simulink model "STEVE_Simulation"  (R2025b)
settings: Solver=ode8  StartTime=0  StopTime=300  FixedStep=0.0001  MaxStep=0.0001  RelTol=1e-3
model workspace (MAT data in the model file):
  op_trim1 = opcond.OperatingReport
  op_trim1.TerminationString_ = 'Operating point specifications were successfully met.'
  op_trim1.OptimizationOutput_.iterations = 3
  op_trim1.OptimizationOutput_.funcCount = 171
  op_trim1.OptimizationOutput_.lssteplength = 1
  op_trim1.OptimizationOutput_.stepsize = 4.63262973918e-09
  op_trim1.OptimizationOutput_.algorithm = 'active-set'
  op_trim1.OptimizationOutput_.firstorderopt = 2.40097601741e-08
  op_trim1.OptimizationOutput_.constrviolation = 8.47716769092e-07
  op_trim1.OptimizationOutput_.message = 'Local minimum found that satisfies the constraints.
    | 
    | Optimization completed because the objective function is non-decreasing in 
    | feasible directions, to within the value of the optimality tolerance,
    | and constraints are satisfied to within the  value of the constraint tolerance.
    | 
    | <stopping criteria details>
    | 
    | Optimization completed: The first-order optimality measure, 2.400976e-08, is less
    | than options.OptimalityTolerance = 1.000000e-06, and the maximum constraint violation,
    | 8.477168e-07,is less than options.ConstraintTolerance = 1.000000e-06.'
  op_trim1.OptimizationOutput_.bestfeasible.x = [4290.04874097; 10725.1258376; 15852.6764872; 0.313155746169; -0.0981866680343; -0.0652604980678; 0.0059055243257; -0.636615168463; 8.14642489212e-06; -0.0176940249338; -0.00155509692213; -9.31199930506e-05; -0.000181100785288; 15.418172162; 0.559389025394; 3.31048087203; -37.2767340788; 1.38336022573; 8.21403291962e-06; 8.22046546553e-06; 8.22180678664e-06; 8.18637735168e-06; 8.165374813e-06; 8.15659926853e-06; 8.21875394544e-06; 8.19540646323e-06; 8.20244331077e-06; 8.1953609355e-06; 8.1983838895e-06; 8.22592390188e-06; 8.20694393928e-06; 8.20085018843e-06; 8.25311843786e-06; 8.2421945992e-06; 4.99999832196; 1.99999584909; 1.99999585143; 4.99999832977; 1.99999587773; 1.999995897; -0.000340053296214]
  op_trim1.OptimizationOutput_.bestfeasible.fval = 0
  op_trim1.OptimizationOutput_.bestfeasible.constrviolation = 8.47716769092e-07
  op_trim1.OptimizationOutput_.bestfeasible.firstorderopt = 2.40097601741e-08
  op_trim1.OptimizationOutput_.progress = {'<font face="monospaced"; size=3><BR>', 'Optimizing to solve for all desired dx/dt=0, x(k+1)-x(k)=0, and y=ydes.<BR>', ' <BR>', '(Maximum Error)  Block<BR>', ' ---------------------------------------------------------<BR>', '(3.86548e-01) STEVE_Simulation/STeVe System Model/Vehicle Dynamics/3DOF to 6DOF/Custom Variable Mass 3dof (Body Axes)<BR>', '(3.86551e-01) STEVE_Simulation/STeVe System Model/Vehicle Dynamics/3DOF to 6DOF/Custom Variable Mass 3dof (Body Axes)<BR>', '(8.47360e-07) STEVE_Simulation/STeVe System Model/Vehicle Dynamics/3DOF to 6DOF/Custom Variable Mass 3dof (Body Axes)<BR>', '(8.47764e-07) STEVE_Simulation/STeVe System Model/Vehicle Dynamics/3DOF to 6DOF/Custom Variable Mass 3dof (Body Axes)<BR>', '(8.47764e-07) STEVE_Simulation/STeVe System Model/Vehicle Dynamics/3DOF to 6DOF/Custom Variable Mass 3dof (Body Axes)<BR>', ' <BR>', 'Operating point specifications were successfully met.<BR>'}
  op_trim1.Model_ = 'STEVE_Simulation'
  op_trim1.States_(1) = opcond.StateReport
  op_trim1.States_(1).Nx_ = 1
  op_trim1.States_(1).Block_ = 'STEVE_Simulation/Environment/Wind/Discrete Wind Gust Model/Distance into
    | gust (x)/Distance into
    | Gust (x)
    | (Limited to gust length d)'
  op_trim1.States_(1).x_ = 1.999995897
  op_trim1.States_(1).SteadyState_ = 0
  op_trim1.States_(1).dxMin_ = -Inf
  op_trim1.States_(1).dxMax_ = Inf
  op_trim1.States_(1).Known_ = 0
  op_trim1.States_(1).Min_ = 0
  op_trim1.States_(1).Max_ = 2
  op_trim1.States_(2) = opcond.StateReport
  op_trim1.States_(2).Nx_ = 1
  op_trim1.States_(2).Block_ = 'STEVE_Simulation/Environment/Wind/Discrete Wind Gust Model/Distance into
    | gust (y)/Distance into
    | Gust (x)
    | (Limited to gust length d)
    | '
  op_trim1.States_(2).x_ = 1.99999587773
  op_trim1.States_(2).SteadyState_ = 0
  op_trim1.States_(2).dxMin_ = -Inf
  op_trim1.States_(2).dxMax_ = Inf
  op_trim1.States_(2).Known_ = 0
  op_trim1.States_(2).Min_ = 0
  op_trim1.States_(2).Max_ = 2
  op_trim1.States_(3) = opcond.StateReport
  op_trim1.States_(3).Nx_ = 1
  op_trim1.States_(3).Block_ = 'STEVE_Simulation/Environment/Wind/Discrete Wind Gust Model/Distance into
    | gust (z)/Distance into
    | Gust (x)
    | (Limited to gust length d)
    | '
  op_trim1.States_(3).x_ = 4.99999832977
  op_trim1.States_(3).SteadyState_ = 0
  op_trim1.States_(3).dxMin_ = -Inf
  op_trim1.States_(3).dxMax_ = Inf
  op_trim1.States_(3).Known_ = 0
  op_trim1.States_(3).Min_ = 0
  op_trim1.States_(3).Max_ = 5
  op_trim1.States_(4) = opcond.StateReport
  op_trim1.States_(4).Nx_ = 1
  op_trim1.States_(4).Block_ = 'STEVE_Simulation/Environment/Wind/Discrete Wind Gust Model1/Distance into
    | gust (x)/Distance into
    | Gust (x)
    | (Limited to gust length d)'
  op_trim1.States_(4).x_ = 1.99999585143
  op_trim1.States_(4).SteadyState_ = 0
  op_trim1.States_(4).dxMin_ = -Inf
  op_trim1.States_(4).dxMax_ = Inf
  op_trim1.States_(4).Known_ = 0
  op_trim1.States_(4).Min_ = 0
  op_trim1.States_(4).Max_ = 2
  op_trim1.States_(5) = opcond.StateReport
  op_trim1.States_(5).Nx_ = 1
  op_trim1.States_(5).Block_ = 'STEVE_Simulation/Environment/Wind/Discrete Wind Gust Model1/Distance into
    | gust (y)/Distance into
    | Gust (x)
    | (Limited to gust length d)
    | '
  op_trim1.States_(5).x_ = 1.99999584909
  op_trim1.States_(5).SteadyState_ = 0
  op_trim1.States_(5).dxMin_ = -Inf
  op_trim1.States_(5).dxMax_ = Inf
  op_trim1.States_(5).Known_ = 0
  op_trim1.States_(5).Min_ = 0
  op_trim1.States_(5).Max_ = 2
  op_trim1.States_(6) = opcond.StateReport
  op_trim1.States_(6).Nx_ = 1
  op_trim1.States_(6).Block_ = 'STEVE_Simulation/Environment/Wind/Discrete Wind Gust Model1/Distance into
    | gust (z)/Distance into
    | Gust (x)
    | (Limited to gust length d)
    | '
  op_trim1.States_(6).x_ = 4.99999832196
  op_trim1.States_(6).SteadyState_ = 0
  op_trim1.States_(6).dxMin_ = -Inf
  op_trim1.States_(6).dxMax_ = Inf
  op_trim1.States_(6).Known_ = 0
  op_trim1.States_(6).Min_ = 0
  op_trim1.States_(6).Max_ = 5
  op_trim1.States_(7) = opcond.StateReport
  op_trim1.States_(7).dx_ = [0; 0]
  op_trim1.States_(7).Nx_ = 2
  op_trim1.States_(7).Block_ = 'STEVE_Simulation/Environment/Wind/Dryden Wind Turbulence Model 
    | (Continuous (+q +r))/Filters on angular rates/Hpgw/pgw_p'
  op_trim1.States_(7).x_ = [8.25311843786e-06; 8.2421945992e-06]
  op_trim1.States_(7).SteadyState_ = [0; 0]
  op_trim1.States_(7).dxMin_ = [-Inf; -Inf]
  op_trim1.States_(7).dxMax_ = [Inf; Inf]
  op_trim1.States_(7).Known_ = [0; 0]
  op_trim1.States_(7).Min_ = [-Inf; -Inf]
  op_trim1.States_(7).Max_ = [Inf; Inf]
  op_trim1.States_(8) = opcond.StateReport
  op_trim1.States_(8).dx_ = [0; 0]
  op_trim1.States_(8).Nx_ = 2
  op_trim1.States_(8).Block_ = 'STEVE_Simulation/Environment/Wind/Dryden Wind Turbulence Model 
    | (Continuous (+q +r))/Filters on angular rates/Hqgw/qgw_p'
  op_trim1.States_(8).x_ = [8.20694393928e-06; 8.20085018843e-06]
  op_trim1.States_(8).SteadyState_ = [0; 0]
  op_trim1.States_(8).dxMin_ = [-Inf; -Inf]
  op_trim1.States_(8).dxMax_ = [Inf; Inf]
  op_trim1.States_(8).Known_ = [0; 0]
  op_trim1.States_(8).Min_ = [-Inf; -Inf]
  op_trim1.States_(8).Max_ = [Inf; Inf]
  op_trim1.States_(9) = opcond.StateReport
  op_trim1.States_(9).dx_ = [0; 0]
  op_trim1.States_(9).Nx_ = 2
  op_trim1.States_(9).Block_ = 'STEVE_Simulation/Environment/Wind/Dryden Wind Turbulence Model 
    | (Continuous (+q +r))/Filters on angular rates/Hrgw/rgw_p'
  op_trim1.States_(9).x_ = [8.1983838895e-06; 8.22592390188e-06]
  op_trim1.States_(9).SteadyState_ = [0; 0]
  op_trim1.States_(9).dxMin_ = [-Inf; -Inf]
  op_trim1.States_(9).dxMax_ = [Inf; Inf]
  op_trim1.States_(9).Known_ = [0; 0]
  op_trim1.States_(9).Min_ = [-Inf; -Inf]
  op_trim1.States_(9).Max_ = [Inf; Inf]
  op_trim1.States_(10) = opcond.StateReport
  op_trim1.States_(10).dx_ = [0; 0]
  op_trim1.States_(10).Nx_ = 2
  op_trim1.States_(10).Block_ = 'STEVE_Simulation/Environment/Wind/Dryden Wind Turbulence Model 
    | (Continuous (+q +r))/Filters on velocities/Hugw(s)/ug_p'
  op_trim1.States_(10).x_ = [8.20244331077e-06; 8.1953609355e-06]
  op_trim1.States_(10).SteadyState_ = [0; 0]
  op_trim1.States_(10).dxMin_ = [-Inf; -Inf]
  op_trim1.States_(10).dxMax_ = [Inf; Inf]
  op_trim1.States_(10).Known_ = [0; 0]
  op_trim1.States_(10).Min_ = [-Inf; -Inf]
  op_trim1.States_(10).Max_ = [Inf; Inf]
  op_trim1.States_(11) = opcond.StateReport
  op_trim1.States_(11).dx_ = [0; 0]
  op_trim1.States_(11).Nx_ = 2
  op_trim1.States_(11).Block_ = 'STEVE_Simulation/Environment/Wind/Dryden Wind Turbulence Model 
    | (Continuous (+q +r))/Filters on velocities/Hvgw(s)/vg_p1'
  op_trim1.States_(11).x_ = [8.165374813e-06; 8.15659926853e-06]
  op_trim1.States_(11).SteadyState_ = [0; 0]
  op_trim1.States_(11).dxMin_ = [-Inf; -Inf]
  op_trim1.States_(11).dxMax_ = [Inf; Inf]
  op_trim1.States_(11).Known_ = [0; 0]
  op_trim1.States_(11).Min_ = [-Inf; -Inf]
  op_trim1.States_(11).Max_ = [Inf; Inf]
  op_trim1.States_(12) = opcond.StateReport
  op_trim1.States_(12).dx_ = [0; 0]
  op_trim1.States_(12).Nx_ = 2
  op_trim1.States_(12).Block_ = 'STEVE_Simulation/Environment/Wind/Dryden Wind Turbulence Model 
    | (Continuous (+q +r))/Filters on velocities/Hvgw(s)/vgw_p2'
  op_trim1.States_(12).x_ = [8.21875394544e-06; 8.19540646323e-06]
  op_trim1.States_(12).SteadyState_ = [0; 0]
  op_trim1.States_(12).dxMin_ = [-Inf; -Inf]
  op_trim1.States_(12).dxMax_ = [Inf; Inf]
  op_trim1.States_(12).Known_ = [0; 0]
  op_trim1.States_(12).Min_ = [-Inf; -Inf]
  op_trim1.States_(12).Max_ = [Inf; Inf]
  op_trim1.States_(13) = opcond.StateReport
  op_trim1.States_(13).dx_ = [0; 0]
  op_trim1.States_(13).Nx_ = 2
  op_trim1.States_(13).Block_ = 'STEVE_Simulation/Environment/Wind/Dryden Wind Turbulence Model 
    | (Continuous (+q +r))/Filters on velocities/Hwgw(s)/wg_p1'
  op_trim1.States_(13).x_ = [8.21403291962e-06; 8.22046546553e-06]
  op_trim1.States_(13).SteadyState_ = [0; 0]
  op_trim1.States_(13).dxMin_ = [-Inf; -Inf]
  op_trim1.States_(13).dxMax_ = [Inf; Inf]
  op_trim1.States_(13).Known_ = [0; 0]
  op_trim1.States_(13).Min_ = [-Inf; -Inf]
  op_trim1.States_(13).Max_ = [Inf; Inf]
  op_trim1.States_(14) = opcond.StateReport
  op_trim1.States_(14).dx_ = [0; 0]
  op_trim1.States_(14).Nx_ = 2
  op_trim1.States_(14).Block_ = 'STEVE_Simulation/Environment/Wind/Dryden Wind Turbulence Model 
    | (Continuous (+q +r))/Filters on velocities/Hwgw(s)/wg_p2'
  op_trim1.States_(14).x_ = [8.22180678664e-06; 8.18637735168e-06]
  op_trim1.States_(14).SteadyState_ = [0; 0]
  op_trim1.States_(14).dxMin_ = [-Inf; -Inf]
  op_trim1.States_(14).dxMax_ = [Inf; Inf]
  op_trim1.States_(14).Known_ = [0; 0]
  op_trim1.States_(14).Min_ = [-Inf; -Inf]
  op_trim1.States_(14).Max_ = [Inf; Inf]
  op_trim1.States_(15) = opcond.StateReport
  op_trim1.States_(15).dx_ = [-1624.62107391; 4290.04874097; 10725.1258376]
  op_trim1.States_(15).Nx_ = 3
  op_trim1.States_(15).Block_ = 'STEVE_Simulation/GuidanceCommands/Transfer Fcn'
  op_trim1.States_(15).x_ = [4290.04874097; 10725.1258376; 15852.6764872]
  op_trim1.States_(15).SteadyState_ = [0; 0; 0]
  op_trim1.States_(15).dxMin_ = [-Inf; -Inf; -Inf]
  op_trim1.States_(15).dxMax_ = [Inf; Inf; Inf]
  op_trim1.States_(15).Known_ = [0; 0; 0]
  op_trim1.States_(15).Min_ = [-Inf; -Inf; -Inf]
  op_trim1.States_(15).Max_ = [Inf; Inf; Inf]
  op_trim1.States_(16) = opcond.StateReport
  op_trim1.States_(16).dx_ = -3.37116243602
  op_trim1.States_(16).Nx_ = 1
  op_trim1.States_(16).Block_ = 'STEVE_Simulation/STeVe System Model/Control System/Classical Upgraded/PID Controller1/Filter/Cont. Filter/Filter'
  op_trim1.States_(16).x_ = -0.00155509692213
  op_trim1.States_(16).SteadyState_ = 0
  op_trim1.States_(16).dxMin_ = -Inf
  op_trim1.States_(16).dxMax_ = Inf
  op_trim1.States_(16).Known_ = 0
  op_trim1.States_(16).Min_ = -Inf
  op_trim1.States_(16).Max_ = Inf
  op_trim1.States_(17) = opcond.StateReport
  op_trim1.States_(17).dx_ = -0.00991390700733
  op_trim1.States_(17).Nx_ = 1
  op_trim1.States_(17).Block_ = 'STEVE_Simulation/STeVe System Model/Control System/Classical Upgraded/PID Controller1/Integrator/Continuous/Integrator'
  op_trim1.States_(17).x_ = -0.0176940249338
  op_trim1.States_(17).SteadyState_ = 0
  op_trim1.States_(17).dxMin_ = -Inf
  op_trim1.States_(17).dxMax_ = Inf
  op_trim1.States_(17).Known_ = 0
  op_trim1.States_(17).Min_ = -Inf
  op_trim1.States_(17).Max_ = Inf
  op_trim1.States_(18) = opcond.StateReport
  op_trim1.States_(18).dx_ = 0.00151513100245
  op_trim1.States_(18).Nx_ = 1
  op_trim1.States_(18).Block_ = 'STEVE_Simulation/STeVe System Model/Control System/Classical Upgraded/PID Controller2/Filter/Cont. Filter/Filter'
  op_trim1.States_(18).x_ = 0.0059055243257
  op_trim1.States_(18).SteadyState_ = 0
  op_trim1.States_(18).dxMin_ = -Inf
  op_trim1.States_(18).dxMax_ = Inf
  op_trim1.States_(18).Known_ = 0
  op_trim1.States_(18).Min_ = -Inf
  op_trim1.States_(18).Max_ = Inf
  op_trim1.States_(19) = opcond.StateReport
  op_trim1.States_(19).dx_ = -0.037481221471
  op_trim1.States_(19).Nx_ = 1
  op_trim1.States_(19).Block_ = 'STEVE_Simulation/STeVe System Model/Control System/Classical Upgraded/PID Controller2/Integrator/Continuous/Integrator'
  op_trim1.States_(19).x_ = -0.0652604980678
  op_trim1.States_(19).SteadyState_ = 0
  op_trim1.States_(19).dxMin_ = -Inf
  op_trim1.States_(19).dxMax_ = Inf
  op_trim1.States_(19).Known_ = 0
  op_trim1.States_(19).Min_ = -Inf
  op_trim1.States_(19).Max_ = Inf
  op_trim1.States_(20) = opcond.StateReport
  op_trim1.States_(20).dx_ = -0.0747869203805
  op_trim1.States_(20).Nx_ = 1
  op_trim1.States_(20).Block_ = 'STEVE_Simulation/STeVe System Model/Control System/Classical Upgraded/PID Controller3/Filter/Cont. Filter/Filter'
  op_trim1.States_(20).x_ = -0.0981866680343
  op_trim1.States_(20).SteadyState_ = 0
  op_trim1.States_(20).dxMin_ = -Inf
  op_trim1.States_(20).dxMax_ = Inf
  op_trim1.States_(20).Known_ = 0
  op_trim1.States_(20).Min_ = -Inf
  op_trim1.States_(20).Max_ = Inf
  op_trim1.States_(21) = opcond.StateReport
  op_trim1.States_(21).dx_ = 0.273198142244
  op_trim1.States_(21).Nx_ = 1
  op_trim1.States_(21).Block_ = 'STEVE_Simulation/STeVe System Model/Control System/Classical Upgraded/PID Controller3/Integrator/Continuous/Integrator'
  op_trim1.States_(21).x_ = 0.313155746169
  op_trim1.States_(21).SteadyState_ = 0
  op_trim1.States_(21).dxMin_ = -Inf
  op_trim1.States_(21).dxMax_ = Inf
  op_trim1.States_(21).Known_ = 0
  op_trim1.States_(21).Min_ = -Inf
  op_trim1.States_(21).Max_ = Inf
  op_trim1.States_(22) = opcond.StateReport
  op_trim1.States_(22).dx_ = -0.000814642489212
  op_trim1.States_(22).Nx_ = 1
  op_trim1.States_(22).Block_ = 'STEVE_Simulation/STeVe System Model/Control System/Classical Upgraded/PID Controller6/Filter/Cont. Filter/Filter'
  op_trim1.States_(22).x_ = 8.14642489212e-06
  op_trim1.States_(22).SteadyState_ = 0
  op_trim1.States_(22).dxMin_ = -Inf
  op_trim1.States_(22).dxMax_ = Inf
  op_trim1.States_(22).Known_ = 0
  op_trim1.States_(22).Min_ = -Inf
  op_trim1.States_(22).Max_ = Inf
  op_trim1.States_(23) = opcond.StateReport
  op_trim1.States_(23).dx_ = -0.133481022202
  op_trim1.States_(23).Nx_ = 1
  op_trim1.States_(23).Block_ = 'STEVE_Simulation/STeVe System Model/Control System/Classical Upgraded/PID Controller6/Integrator/Continuous/Integrator'
  op_trim1.States_(23).x_ = -0.636615168463
  op_trim1.States_(23).SteadyState_ = 0
  op_trim1.States_(23).dxMin_ = -Inf
  op_trim1.States_(23).dxMax_ = Inf
  op_trim1.States_(23).Known_ = 0
  op_trim1.States_(23).Min_ = -Inf
  op_trim1.States_(23).Max_ = Inf
  op_trim1.States_(24) = opcond.StateReport
  op_trim1.States_(24).dx_ = 3.05199662227
  op_trim1.States_(24).Nx_ = 1
  op_trim1.States_(24).Block_ = 'STEVE_Simulation/STeVe System Model/Vehicle Dynamics/3DOF to 6DOF/Custom Variable Mass 3dof
    | (Body Axes)'
  op_trim1.States_(24).StateName_ = 'u'
  op_trim1.States_(24).x_ = 15.418172162
  op_trim1.States_(24).SteadyState_ = 0
  op_trim1.States_(24).dxMin_ = -Inf
  op_trim1.States_(24).dxMax_ = Inf
  op_trim1.States_(24).Known_ = 0
  op_trim1.States_(24).Min_ = -Inf
  op_trim1.States_(24).Max_ = Inf
  op_trim1.States_(25) = opcond.StateReport
  op_trim1.States_(25).dx_ = 1.82984252685
  op_trim1.States_(25).Nx_ = 1
  op_trim1.States_(25).Block_ = 'STEVE_Simulation/STeVe System Model/Vehicle Dynamics/3DOF to 6DOF/Custom Variable Mass 3dof
    | (Body Axes)'
  op_trim1.States_(25).StateName_ = 'w'
  op_trim1.States_(25).x_ = 0.559389025394
  op_trim1.States_(25).SteadyState_ = 0
  op_trim1.States_(25).dxMin_ = -Inf
  op_trim1.States_(25).dxMax_ = Inf
  op_trim1.States_(25).Known_ = 0
  op_trim1.States_(25).Min_ = -Inf
  op_trim1.States_(25).Max_ = Inf
  op_trim1.States_(26) = opcond.StateReport
  op_trim1.States_(26).dx_ = 3.42262162857
  op_trim1.States_(26).Nx_ = 1
  op_trim1.States_(26).Block_ = 'STEVE_Simulation/STeVe System Model/Vehicle Dynamics/3DOF to 6DOF/Custom Variable Mass 3dof
    | (Body Axes)'
  op_trim1.States_(26).StateName_ = 'Xe'
  op_trim1.States_(26).x_ = 3.31048087203
  op_trim1.States_(26).SteadyState_ = 0
  op_trim1.States_(26).dxMin_ = -Inf
  op_trim1.States_(26).dxMax_ = Inf
  op_trim1.States_(26).Known_ = 0
  op_trim1.States_(26).Min_ = -Inf
  op_trim1.States_(26).Max_ = Inf
  op_trim1.States_(27) = opcond.StateReport
  op_trim1.States_(27).dx_ = -15.0438894601
  op_trim1.States_(27).Nx_ = 1
  op_trim1.States_(27).Block_ = 'STEVE_Simulation/STeVe System Model/Vehicle Dynamics/3DOF to 6DOF/Custom Variable Mass 3dof
    | (Body Axes)'
  op_trim1.States_(27).StateName_ = 'Ze'
  op_trim1.States_(27).x_ = -37.2767340788
  op_trim1.States_(27).SteadyState_ = 0
  op_trim1.States_(27).dxMin_ = -Inf
  op_trim1.States_(27).dxMax_ = Inf
  op_trim1.States_(27).Known_ = 0
  op_trim1.States_(27).Min_ = -Inf
  op_trim1.States_(27).Max_ = Inf
  op_trim1.States_(28) = opcond.StateReport
  op_trim1.States_(28).dx_ = 8.47764429975e-07
  op_trim1.States_(28).Nx_ = 1
  op_trim1.States_(28).Block_ = 'STEVE_Simulation/STeVe System Model/Vehicle Dynamics/3DOF to 6DOF/Custom Variable Mass 3dof
    | (Body Axes)'
  op_trim1.States_(28).StateName_ = 'q'
  op_trim1.States_(28).SteadyState_ = 1
  op_trim1.States_(28).dxMin_ = -Inf
  op_trim1.States_(28).dxMax_ = Inf
  op_trim1.States_(28).Known_ = 1
  op_trim1.States_(28).Min_ = -Inf
  op_trim1.States_(28).Max_ = Inf
  op_trim1.States_(29) = opcond.StateReport
  op_trim1.States_(29).Nx_ = 1
  op_trim1.States_(29).Block_ = 'STEVE_Simulation/STeVe System Model/Vehicle Dynamics/3DOF to 6DOF/Custom Variable Mass 3dof
    | (Body Axes)'
  op_trim1.States_(29).StateName_ = 'theta'
  op_trim1.States_(29).x_ = 1.38336022573
  op_trim1.States_(29).SteadyState_ = 1
  op_trim1.States_(29).dxMin_ = -Inf
  op_trim1.States_(29).dxMax_ = Inf
  op_trim1.States_(29).Known_ = 0
  op_trim1.States_(29).Min_ = -Inf
  op_trim1.States_(29).Max_ = Inf
  op_trim1.States_(30) = opcond.StateReport
  op_trim1.States_(30).dx_ = -3.39724258746
  op_trim1.States_(30).Nx_ = 1
  op_trim1.States_(30).Block_ = 'STEVE_Simulation/STeVe System Model/Vehicle Dynamics/RocketEngineActuators/Delay'
  op_trim1.States_(30).x_ = -0.000340053296214
  op_trim1.States_(30).Ts_ = [0.0001 0]
  op_trim1.States_(30).SampleType_ = 'DSTATE'
  op_trim1.States_(30).SteadyState_ = 0
  op_trim1.States_(30).dxMin_ = -Inf
  op_trim1.States_(30).dxMax_ = Inf
  op_trim1.States_(30).Known_ = 0
  op_trim1.States_(30).Min_ = -Inf
  op_trim1.States_(30).Max_ = Inf
  op_trim1.States_(31) = opcond.StateReport
  op_trim1.States_(31).dx_ = [-0.000181100785288; -0.936056601197]
  op_trim1.States_(31).Nx_ = 2
  op_trim1.States_(31).Block_ = 'STEVE_Simulation/STeVe System Model/Vehicle Dynamics/RocketEngineActuators/Servo/Integrator,
    | Second-Order
    | Limited'
  op_trim1.States_(31).x_ = [-9.31199930506e-05; -0.000181100785288]
  op_trim1.States_(31).SteadyState_ = [0; 0]
  op_trim1.States_(31).dxMin_ = [-Inf; -Inf]
  op_trim1.States_(31).dxMax_ = [Inf; Inf]
  op_trim1.States_(31).Known_ = [0; 0]
  op_trim1.States_(31).Min_ = [-Inf; -Inf]
  op_trim1.States_(31).Max_ = [Inf; Inf]
undefined symbols (not defined in the file): a_gyro_fast, Actuators, AeroData, b_gyro_fast, C_inner_launch_d_Kd, C_inner_launch_d_Ki, C_inner_launch_d_Kp, C_inner_maxQ_d_Kd, C_inner_maxQ_d_Ki, C_inner_maxQ_d_Kp, C_inner_maxQ_d_Tf, C_outer_launch_d_Kd, C_outer_launch_d_Ki, C_outer_launch_d_Kp, C_outer_launch_d_N, C_outer_maxQ_d_Kd, C_outer_maxQ_d_Ki, C_outer_maxQ_d_Kp, dspblkCoreblockFVToolHelper, F, fractalcoef, fs_filter, fs_gyro, gcbh, Initial, K_gains, Light, max_q_margin, MIL, PrelookupData, Ref_Area, rocket_length, RocketAeroPhysical, time_vector, timeStep, Ts_inner, Ts_outer, wn_ramp
libraries: simulink x14, simulink_extras x11, slpidlib x10, aerolibwind2 x3, aerolibasang x3, aerolibtransform2 x2, aerolibatmos2 x1, sensorgpslib x1, mspsensorlib x1, aerolibconvert2 x1, aerolibactuator x1
(part 1 of 3)
settings Model: SimulationMode=accelerator  ExtModeTrigDuration=2  Creator=jonno  LastModifiedBy=jonno
settings SolverCC: AutoInsertRateTranBlk=on
settings DataIOCC: ExternalInput=getinputstruct(op_trim1)  InitialState=getstatestruct(op_trim1)  SaveFormat=StructureWithTime
settings OptimizationCC: BlockReduction=off  BufferReuse=off
settings DebuggingCC: AlgebraicLoopMsg=none
settings HardwareCC: ProdBitPerLong=64.0  ProdHWDeviceType=Apple->ARM64
settings RTWCC: BuildConfiguration=Faster Runs
settings GRTTargetCC: RTWCAPISignals=on  RTWCAPIParams=on
settings ExplorerConfigSet: SimMechanicsOpenEditorOnUpdate=off

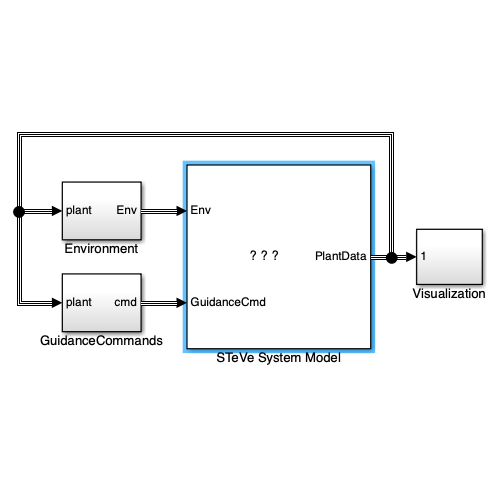
[thumbnail: Simulink's stored preview of the top-level diagram]
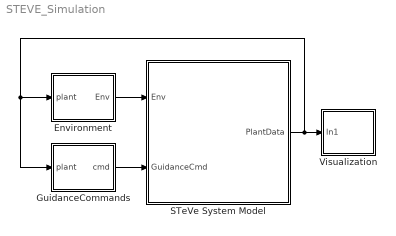
== system STEVE_Simulation ==
  Environment : Subsystem
  GuidanceCommands : Subsystem
  STeVe System Model : Subsystem
      mask Display: image('/Users/jonno/MATLAB-Drive/masters-rocket-control-repository/simulation/docs/images/steve.png', [65 - (50 * (187 / 1041)), 0, 140 * (187 / 1041), 140])
  Visualization : Subsystem
  wires:
  GuidanceCommands/1(cmd) -> STeVe System Model/2(GuidanceCmd)
  Environment/1(Env) -> STeVe System Model/1(Env)
  STeVe System Model/1(PlantData) -> GuidanceCommands/1(plant), Environment/1(plant), Visualization/1(In1)

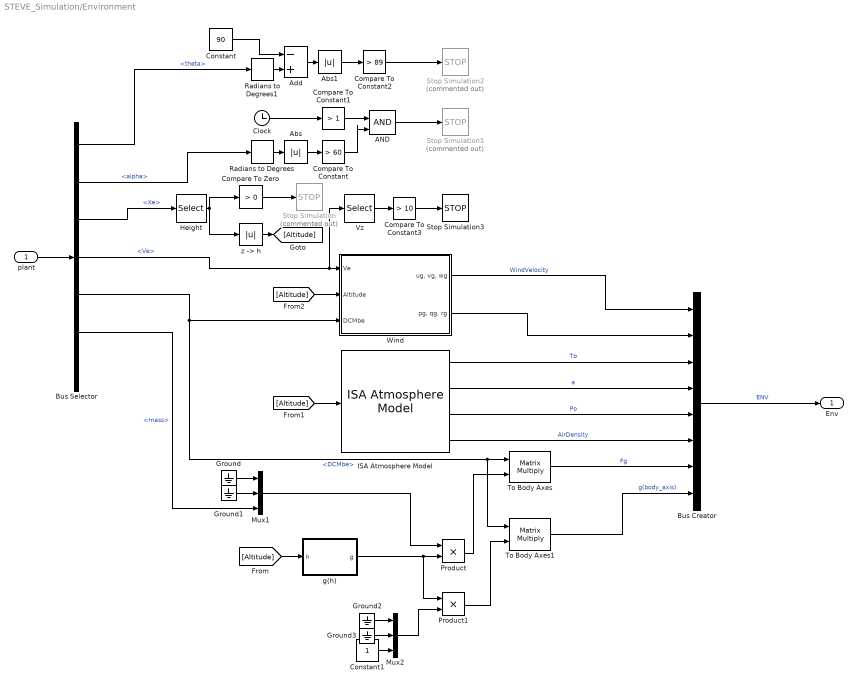
== system STEVE_Simulation/Environment ==
  plant : Inport
  AND : Logic  IconShape=distinctive  AllPortsSameDT=off  OutDataTypeStr=boolean
  Abs : Abs  SaturateOnIntegerOverflow=off
  Abs1 : Abs  SaturateOnIntegerOverflow=off
  Add : Sum  Inputs=-+
  Bus Creator : BusCreator  Inputs=8
  Bus Selector : BusSelector  OutputSignals=body angles.theta,alpha,Xe,Ve,DCMbe,mass,lat
  Clock : Clock
  Compare To Constant : simulink/Logic and Bit Operations/Compare To Constant  relop=>  const=60  OutDataTypeStr=boolean
  Compare To Constant1 : simulink/Logic and Bit Operations/Compare To Constant  relop=>  const=1  OutDataTypeStr=boolean
  Compare To Constant2 : simulink/Logic and Bit Operations/Compare To Constant  relop=>  const=89  OutDataTypeStr=boolean
  Compare To Constant3 : simulink/Logic and Bit Operations/Compare To Constant  relop=>  const=10  OutDataTypeStr=boolean
  Compare To Zero : simulink/Logic and Bit Operations/Compare To Zero  relop=>  OutDataTypeStr=boolean
  Constant : Constant  Value=90
  Constant1 : Constant
  Ground{,1..3} (4 alike) : Ground
  Height : Selector  IndexMode=Zero-based  InputPortWidth=3  IndexOptions=Index vector (dialog)  Indices=2  OutputSizes=1
  ISA Atmosphere Model : aerolibatmos2/ISA Atmosphere Model  useExtended=on  action=None  custom=off  viscosityOut=off  g=9.80665  gamma=1.4  R=287.0531  L=0.0065  h_trop=11000  h_strat=20000  rho0=1.225  P0=101325  T0=288.15  h0=0  S=110.4  Tref=273.15  muref=1.716e-5
  Mux1 : Mux  Inputs=3
  Mux2 : Mux  Inputs=3
  Product : Product
  Product1 : Product
  Radians to Degrees : simulink_extras/Transformations/Radians to Degrees
  Radians to Degrees1 : simulink_extras/Transformations/Radians to Degrees
  Stop Simulation : Stop  Commented=on
  Stop Simulation1 : Stop  Commented=on
  Stop Simulation2 : Stop  Commented=on
  Stop Simulation3 : Stop
  To Body Axes : Product  Multiplication=Matrix(*)
  To Body Axes1 : Product  Multiplication=Matrix(*)
  Vz : Selector  IndexMode=Zero-based  InputPortWidth=3  IndexOptions=Index vector (dialog)  Indices=2  OutputSizes=1
  Wind : Subsystem
  g(h) : MATLAB Function  TreatAsAtomicUnit=on
  "z -> h" : Abs  SaturateOnIntegerOverflow=off
  Env : Outport
  wires:
  plant/1 -> Bus Selector/1
  Bus Creator/1 -> Env/1  "ENV"
  Bus Selector/3 -> Height/1  "<Xe>"
  Height/1 -> "z -> h"/1, Compare To Zero/1
  "z -> h"/1 -> [Altitude]
  Bus Selector/6 -> Mux1/3  "<mass>"
  Ground/1 -> Mux1/1
  Ground1/1 -> Mux1/2
  Bus Selector/5 -> Wind/3(DCMbe), To Body Axes1/1, To Body Axes/1  "<DCMbe>"
  [Altitude] -> ISA Atmosphere Model/1
  To Body Axes/1 -> Bus Creator/7  "Fg"
  ISA Atmosphere Model/4 -> Bus Creator/6  "AirDensity"
  ISA Atmosphere Model/3 -> Bus Creator/5  "Po"
  ISA Atmosphere Model/2 -> Bus Creator/4  "a"
  ISA Atmosphere Model/1 -> Bus Creator/3  "To"
  Bus Selector/4 -> Vz/1, Wind/1(Ve)  "<Ve>"
  [Altitude] -> Wind/2(Altitude)
  Wind/2("pg, qg, rg") -> Bus Creator/2
  Mux1/1 -> Product/1
  Product/1 -> To Body Axes/2
  [Altitude] -> g(h)/1(h)
  g(h)/1(g) -> Product1/1, Product/2
  Wind/1("ug, vg, wg") -> Bus Creator/1  "WindVelocity"
  Bus Selector/2 -> Radians to Degrees/1  "<alpha>"
  Compare To Zero/1 -> Stop Simulation/1
  AND/1 -> Stop Simulation1/1
  Compare To Constant/1 -> AND/2
  Compare To Constant1/1 -> AND/1
  Clock/1 -> Compare To Constant1/1
  Radians to Degrees/1 -> Abs/1
  Abs/1 -> Compare To Constant/1
  Bus Selector/1 -> Radians to Degrees1/1  "<theta>"
  Radians to Degrees1/1 -> Add/2
  Constant/1 -> Add/1
  Add/1 -> Abs1/1
  Abs1/1 -> Compare To Constant2/1
  Compare To Constant2/1 -> Stop Simulation2/1
  Ground2/1 -> Mux2/1
  Ground3/1 -> Mux2/2
  Constant1/1 -> Mux2/3
  Mux2/1 -> Product1/2
  Product1/1 -> To Body Axes1/2
  To Body Axes1/1 -> Bus Creator/8  "g(body_axis)"
  Compare To Constant3/1 -> Stop Simulation3/1
  Vz/1 -> Compare To Constant3/1

== system STEVE_Simulation/GuidanceCommands ==
  plant : Inport
  Bus Creator : BusCreator  Inputs=3
  Constant : Constant  Value=90
  Degrees to Radians : simulink_extras/Transformations/Degrees to Radians
  Rate Limiter : RateLimiter  RisingSlewLimit=2000/60  FallingSlewLimit=-0.5  SampleTimeMode=inherited
  Rate Limiter2 : RateLimiter  RisingSlewLimit=0.5  FallingSlewLimit=-0.5  SampleTimeMode=inherited
  Step : Step  After=2000  SampleTime=0
  ThrottleCmd %1 : Step  Time=Actuators.Engine.BurnTime  Before=1  After=0.0001  SampleTime=0  VectorParams1D=off
  cmd : Outport
  wires:
  Bus Creator/1 -> cmd/1  "CMD"
  Degrees to Radians/1 -> Bus Creator/2  "ThetaCmd"
  ThrottleCmd %1/1 -> Rate Limiter2/1  "ThrottleCmd"
  Rate Limiter2/1 -> Bus Creator/1  "ThrottleCmd"
  Constant/1 -> Degrees to Radians/1
  Step/1 -> Rate Limiter/1
  Rate Limiter/1 -> Bus Creator/3  "Xe_Cmd"

== system STEVE_Simulation/STeVe System Model ==
  Env : Inport
  GuidanceCmd : Inport  Port=2
  Control System : Subsystem
  Env1 : InportShadow
  State Estimator : Subsystem
  Vehicle Dynamics : Subsystem
  PlantData : Outport
  wires:
  Env/1 -> Vehicle Dynamics/1(Env)
  Vehicle Dynamics/1(PlantData) -> State Estimator/2(Plant), Control System/3(PlantData), PlantData/1  "Plant"
  Control System/1(ActCmd) -> Vehicle Dynamics/2(ActCmd)
  GuidanceCmd/1 -> Control System/1(GuidanceCommandBus)
  Env1/1 -> State Estimator/1(Env)
  State Estimator/1(Sensors) -> Control System/2(Sensors)

== system STEVE_Simulation/Visualization ==
  In1 : Inport
  Add Constant : Bias  Bias=-90  SaturateOnIntegerOverflow=off
  Bus Selector : BusSelector  OutputSignals=Xe,body angles.theta
  Demux : Demux  Outputs=3
  Multiply : Gain  Gain=-1
  Radians to Degrees : simulink_extras/Transformations/Radians to Degrees
  Scope : Scope
      settings: ActiveDisplayYMinimum=-14.168364272787372  ActiveDisplayYMaximum=31.525148324728235  DataLoggingVariableName=ScopeData7
  XY Graph : Record  NumPorts=2.0  FileSettingsInternal="{\"entries\":[{\"content\":{\"excelSettings\":{\"content\":{},\"type\":\"Streamout.ExcelSettings\"},\"parquetSettings\":{\"content\":{},\"type\":\"Streamout.ParquetSettings\"}},\"type\":\"Streamout.FileSettingStorage\",\"uuid\":\"\"}],\"packageUris\":[\"http:\\/\\/schema.mathworks.com\\/mf0\\/streamout_blocks\\/R2020a\"],\"version\":\"1.0\"}"  FrameSettings=[0, 0]  Layout=[1 1]  SignalsInternal="{\"entries\":[{\"content\":{\"signals\":[{\"content\":{\"blockPath\":[],\"dimensions\":[1],\"domain\":\"\",\"lineColor\":\"#4dbeee\",\"lineWidth\":2,\"port\":1,\"sid\":[\"\"],\"signalID\":1,\"signalName\":\"Demux:1\"},\"type\":\"RecordBlkView.Signal\",\"uuid\":\"\"},{\"content\":{\"blockPath\":[],\"dimensions\":[1],\"domain\":\"\",\"lineColor\":\"#a2142f\",\"lineWidth\":2,\"port\":2,\"sid\":[\"\"],\"signalID\":2,\"signalName\":\"Multiply\"},\"type\":\"RecordBlkView.Signal\",\"uuid\":\"\"}]},\"type\":\"RecordBlkView.InputSignals\",\"uuid\":\"\"}],\"packageUris\":[\"http:\\/\\/schema.mathworks.com\\/mf0\\/streamout_blocks\\/R2020a\"],\"version\":\"1.0\"}"  VisualizationBindings="{\"xyplotplugin\":{\"info\":[{\"series\":[],\"subplotID\":1}]}}"  CompatibilityTag=XY
  wires:
  In1/1 -> Bus Selector/1
  Bus Selector/1 -> Demux/1  "<Xe>"
  Multiply/1 -> XY Graph/2
  Demux/3 -> Multiply/1
  Demux/1 -> XY Graph/1
  Bus Selector/2 -> Radians to Degrees/1  "<theta>"
  Radians to Degrees/1 -> Add Constant/1
  Add Constant/1 -> Scope/1  "theta_variation_deg"

== system STEVE_Simulation/Environment/Wind ==
  Ve : Inport
  Altitude : Inport  Port=2
  DCMbe : Inport  Port=3
  Discrete Wind Gust Model : aerolibwind2/Discrete Wind Gust Model  units=Metric (MKS)  Gx=on  Gy=off  Gz=off  t_0=1  d_m=[50 10 10]  v_m=[30 0 0]
  Dot Product : DotProduct  OutDataTypeStr=Inherit: Inherit via internal rule
  Dryden Wind Turbulence Model (Continuous (+q +r)) : aerolibwind2/Dryden Wind Turbulence Model  (Continuous (+q -r))  units=Metric (MKS)  spec=MIL-F-8785C  model=Continuous Dryden (+q +r)  W20=15  Wdeg=0  TurbProb=10^-2 - Light  L_high=533.4  Wingspan=10  ts=0.1  Seed=[23341 23342 23343 23344]  T_on=off
      settings: LibrarySourceBlock=|
      | aerolibwind2/Dryden Wind Turbulence Model
      | (Continuous (+q +r))
  Multiply : Gain
  Multiply1 : Gain
  Multiply2 : Gain  Gain=0
  Scope : Scope
      settings: ActiveDisplayYMinimum=-3.4473346269998206  ActiveDisplayYMaximum=16.02681366587808  DataLoggingVariableName=ScopeData5
  Sum : Sum  Inputs=+++
  Wind Shear Model : aerolibwind2/Wind Shear Model  units=Metric (MKS)  phase=Category C - Terminal Flight Phase  W_20=Wind.shear  Wdeg=90
  vt : Sqrt
  "ug, vg, wg" : Outport
  "pg, qg, rg" : Outport  Port=2
  tag scope: Airspeed=global
  wires:
  Ve/1 -> Dot Product/2, Dot Product/1
  Dot Product/1 -> vt/1
  vt/1 -> [Airspeed]
  DCMbe/1 -> [DCMbe]
  [Altitude] -> Wind Shear Model/1
  [DCMbe] -> Wind Shear Model/2
  [Altitude] -> Dryden Wind Turbulence Model (Continuous (+q +r))/1
  [DCMbe] -> Dryden Wind Turbulence Model (Continuous (+q +r))/3
  [Airspeed] -> Dryden Wind Turbulence Model (Continuous (+q +r))/2
  [Airspeed] -> Discrete Wind Gust Model/1
  Sum/1 -> "ug, vg, wg"/1  "WindVelocity"
  Dryden Wind Turbulence Model (Continuous (+q +r))/2 -> "pg, qg, rg"/1  "WindAngularRates"
  Altitude/1 -> [Altitude]
  Multiply/1 -> Sum/3, Scope/1
  Wind Shear Model/1 -> Multiply2/1
  Dryden Wind Turbulence Model (Continuous (+q +r))/1 -> Multiply1/1
  Multiply1/1 -> Sum/2
  Multiply2/1 -> Sum/1
  Discrete Wind Gust Model/1 -> Multiply/1

== system STEVE_Simulation/STeVe System Model/Control System ==
  GuidanceCommandBus : Inport
  Sensors : Inport  Port=2
  PlantData : Inport  Port=3
  Classical Upgraded : Subsystem  Commented=on
  Classical Upgraded1 : Subsystem  Commented=on
  Classical Upgraded2 : Subsystem
  ControlSystem Classical : Subsystem  Commented=on
  GuidanceCommandBus1 : InportShadow
  LQR1 : Subsystem  Commented=on
  PlantData1 : InportShadow  Port=3
  Sensors1 : InportShadow  Port=2
  ActCmd : Outport
  wires:
  PlantData/1 -> Classical Upgraded/1(PlantData)
  GuidanceCommandBus/1 -> Classical Upgraded/3(CMD)
  Classical Upgraded/1(Cmd Out) -> ?
  Sensors/1 -> Classical Upgraded/2(Sensors)
  Classical Upgraded2/1(Cmd Out) -> ActCmd/1
  GuidanceCommandBus1/1 -> Classical Upgraded2/3(CMD)
  Sensors1/1 -> Classical Upgraded2/2(Sensors)
  PlantData1/1 -> Classical Upgraded2/1(PlantData)

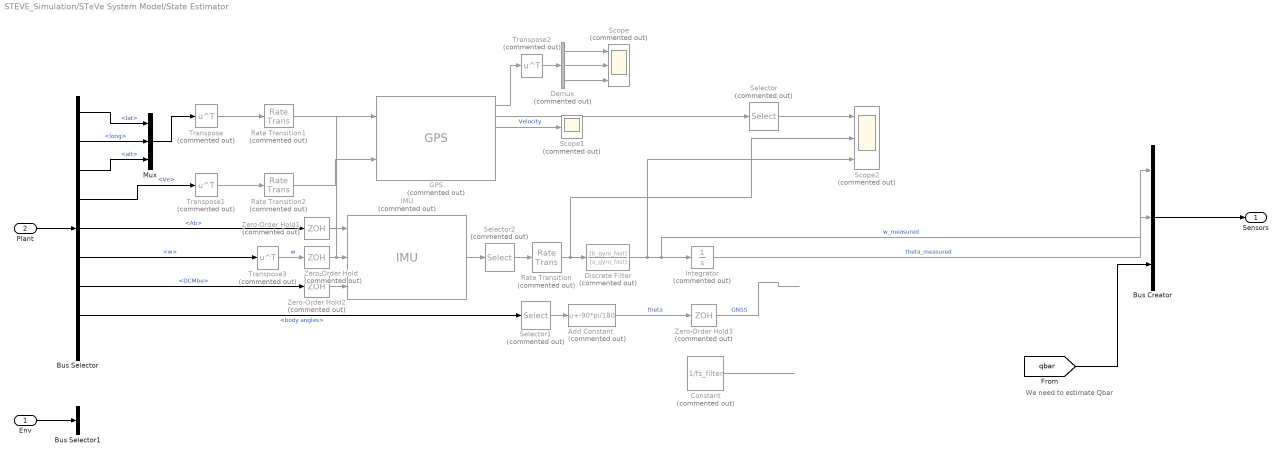
== system STEVE_Simulation/STeVe System Model/State Estimator ==
  note: We need to estimate Qbar
  Env : Inport
  Plant : Inport  Port=2
  Add Constant : Bias  Commented=on  Bias=-90*pi/180  SaturateOnIntegerOverflow=off
  Bus Creator : BusCreator  Inputs=3
  Bus Selector : BusSelector  OutputSignals=lat,long,alt,Ve,Ab,w,DCMbe,body angles,Xe
  Bus Selector1 : BusSelector  OutputSignals=g(body_axis),AirDensity
  Constant : Constant  Commented=on  Value=1/fs_filter
  Demux : Demux  Commented=on  Outputs=3
  Discrete Filter : DiscreteFilter  Commented=on  LoadFcn=dspblkCoreblockFVToolHelper(gcbh,'load');  Numerator=[b_gyro_fast]  Denominator=[a_gyro_fast]
      settings: CopyFcn=dspblkCoreblockFVToolHelper(gcbh,'copy');  DeleteFcn=dspblkCoreblockFVToolHelper(gcbh,'close');  ModelCloseFcn=dspblkCoreblockFVToolHelper(gcbh,'close');  PreSaveFcn=dspblkCoreblockFVToolHelper(gcbh,'presave');  PostSaveFcn=dspblkCoreblockFVToolHelper(gcbh,'postsave');  CloseFcn=dspblkCoreblockFVToolHelper(gcbh,'close');
  GPS : sensorgpslib/GPS  Commented=on  DispRefFrame=NED  PositionInputFormat=Local  ReferenceLocation=[ 0, 0, 0 ]  HorizontalPositionAccuracy=1.5  VerticalPositionAccuracy=3  VelocityAccuracy=0.1  DecayFactor=0.999  SeedDouble=67  SimulateUsing=Interpreted execution
  IMU : mspsensorlib/IMU  Commented=on  DispRefFrame=NED  TemperaturePort=off  Temperature=25  MagneticFieldPort=off  MagneticFieldNED=[ 27.5550, -2.4169, -16.0849 ]  MagneticFieldENU=[ -2.4169, 27.5550, 16.0849 ]  SeedDouble=67  SimulateUsing=Interpreted execution  AccelParamsMeasurementRange=Inf  AccelParamsResolution=0  AccelParamsConstantBias=[ 0, 0, 0 ]  AccelParamsAxesMisalignment=[ 100, 0, 0; 0, 100, 0; 0, 0, 100 ]  AccelParamsNoiseDensity=[ 0, 0, 0 ]  AccelParamsBiasInstability=[ 0, 0, 0 ]  AccelParamsBiasInstabilityNumerator=fractalcoef().Numerator  AccelParamsBiasInstabilityDenominator=fractalcoef().Denominator  AccelParamsRandomWalk=[ 0, 0, 0 ]  AccelParamsNoiseType=double-sided  AccelParamsTemperatureBias=[ 0, 0, 0 ]  AccelParamsTemperatureScaleFactor=[ 0, 0, 0 ]  GyroParamsMeasurementRange=400*pi/180  GyroParamsResolution=((2^-14 )* pi/180)  GyroParamsConstantBias=[4.848e-6, 4.848e-6, 4.848e-6]  GyroParamsAxesMisalignment=[100, 0.1, 0.1; 0.1, 100, 0.1; 0.1, 0.1, 100]  GyroParamsAccelerationBias=[ 3.457e-6, 3.457e-6, 3.457e-6]  GyroParamsNoiseDensity=[ 4.36e-5, 4.36e-5, 4.36e-5]  GyroParamsBiasInstability=[ 2.424e-6,2.424e-6 , 2.424e-6 ]  GyroParamsBiasInstabilityNumerator=fractalcoef().Numerator  GyroParamsBiasInstabilityDenominator=fractalcoef().Denominator  GyroParamsRandomWalk=[ 0, 0, 0 ]  GyroParamsNoiseType=double-sided  GyroParamsTemperatureBias=[ 0, 0, 0 ]  GyroParamsTemperatureScaleFactor=[ 0, 0, 0 ]  MagParamsMeasurementRange=Inf  MagParamsResolution=0  MagParamsConstantBias=[ 0, 0, 0 ]  MagParamsAxesMisalignment=[ 100, 0, 0; 0, 100, 0; 0, 0, 100 ]  MagParamsNoiseDensity=[ 0, 0, 0 ]  MagParamsBiasInstability=[ 0, 0, 0 ]  MagParamsBiasInstabilityNumerator=fractalcoef().Numerator  MagParamsBiasInstabilityDenominator=fractalcoef().Denominator  MagParamsRandomWalk=[ 0, 0, 0 ]  MagParamsNoiseType=double-sided  MagParamsTemperatureBias=[ 0, 0, 0 ]  MagParamsTemperatureScaleFactor=[ 0, 0, 0 ]
  Integrator : Integrator  Commented=on
  Mux : Mux  Inputs=3
  Rate Transition : RateTransition  Commented=on  OutPortSampleTime=1/fs_filter
  Rate Transition1 : RateTransition  Commented=on  OutPortSampleTime=1/25
  Rate Transition2 : RateTransition  Commented=on  OutPortSampleTime=1/25
  Scope : Scope  Commented=on  NumInputPorts=3
      settings: ActiveDisplayYMinimum=-1.1757474819567659E-5  ActiveDisplayYMaximum=2.710364657556593E-5  DataLoggingVariableName=ScopeData8
  Scope1 : Scope  Commented=on
      settings: ActiveDisplayYMinimum=-1  ActiveDisplayYMaximum=1  DataLoggingVariableName=ScopeData10
  Scope2 : Scope  Commented=on  NumInputPorts=3
      settings: ActiveDisplayYMinimum=-0.0199355306051449  ActiveDisplayYMaximum=0.0038603806688270858  DataLoggingVariableName=ScopeData11
  Selector : Selector  Commented=on  InputPortWidth=3  IndexOptions=Index vector (dialog)  Indices=[2]  OutputSizes=1
  Selector1 : Selector  Commented=on  InputPortWidth=3  IndexOptions=Index vector (dialog)  Indices=[2]  OutputSizes=1
  Selector2 : Selector  Commented=on  InputPortWidth=3  IndexOptions=Index vector (dialog)  Indices=[2]  OutputSizes=1
  Transpose{,1..3} (4 alike) : Math  Commented=on  Operator=transpose
  Zero-Order Hold : ZeroOrderHold  Commented=on  SampleTime=1/fs_gyro
  Zero-Order Hold1 : ZeroOrderHold  Commented=on  SampleTime=1/fs_gyro
  Zero-Order Hold2 : ZeroOrderHold  Commented=on  SampleTime=1/fs_gyro
  Zero-Order Hold3 : ZeroOrderHold  Commented=on
  Sensors : Outport
  wires:
  Plant/1 -> Bus Selector/1
  Bus Selector/5 -> Zero-Order Hold1/1  "<Ab>"
  Bus Selector/6 -> Transpose3/1  "<w>"
  Env/1 -> Bus Selector1/1
  Bus Creator/1 -> Sensors/1
  Transpose3/1 -> Zero-Order Hold/1  "w"
  Bus Selector/7 -> Zero-Order Hold2/1  "<DCMbe>"
  Integrator/1 -> Bus Creator/2  "theta_measured"
  Discrete Filter/1 -> Scope2/3, Bus Creator/1, Integrator/1  "w_measured"
  Selector2/1 -> Rate Transition/1
  [qbar] -> Bus Creator/3
  IMU/2 -> Selector2/1
  Rate Transition/1 -> Scope2/2, Discrete Filter/1
  Zero-Order Hold/1 -> Selector/1, IMU/2
  Zero-Order Hold1/1 -> IMU/1
  Zero-Order Hold2/1 -> IMU/3
  Bus Selector/8 -> Selector1/1  "<body angles>"
  Zero-Order Hold3/1 -> ?  "GNSS"
  Selector1/1 -> Add Constant/1
  Add Constant/1 -> Zero-Order Hold3/1  "theta"
  Constant/1 -> ?
  Mux/1 -> Transpose/1
  Bus Selector/1 -> Mux/1  "<lat>"
  Bus Selector/2 -> Mux/2  "<long>"
  Bus Selector/3 -> Mux/3  "<alt>"
  Transpose/1 -> Rate Transition1/1
  Rate Transition1/1 -> GPS/1
  Bus Selector/4 -> Transpose1/1  "<Ve>"
  Transpose1/1 -> Rate Transition2/1
  Rate Transition2/1 -> GPS/2
  GPS/2 -> Scope1/1  "Velocity"
  GPS/1 -> Transpose2/1
  Demux/1 -> Scope/1
  Demux/2 -> Scope/2
  Demux/3 -> Scope/3
  Transpose2/1 -> Demux/1
  Selector/1 -> Scope2/1

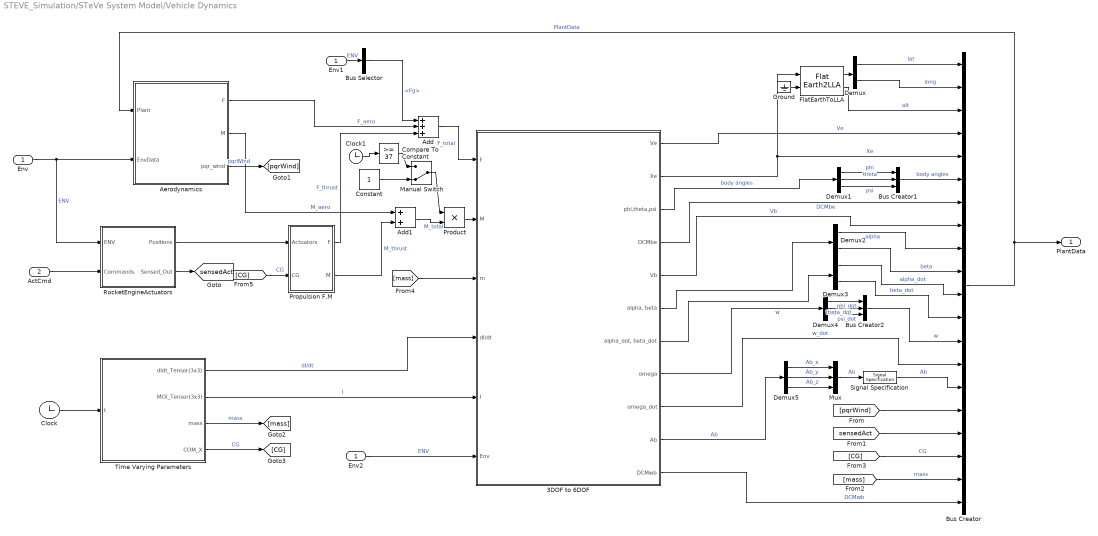
== system STEVE_Simulation/STeVe System Model/Vehicle Dynamics ==
  Env : Inport
  ActCmd : Inport  Port=2
  3DOF to 6DOF : Subsystem
  Add : Sum  Inputs=+++
  Add1 : Sum
  Aerodynamics : Subsystem
  Bus Creator : BusCreator  Inputs=20
  Bus Creator1 : BusCreator  Inputs=3
  Bus Creator2 : BusCreator  Inputs=3
  Bus Selector : BusSelector  OutputSignals=Fg
  Clock : Clock
  Clock1 : Clock
  Compare To Constant : simulink/Logic and Bit Operations/Compare To Constant  relop=>=  const=37  OutDataTypeStr=boolean
  Constant : Constant
  Demux : Demux  Outputs=2
  Demux1 : Demux  Outputs=3
  Demux2 : Demux  Outputs=2
  Demux3 : Demux  Outputs=2
  Demux4 : Demux  Outputs=3
  Demux5 : Demux  Outputs=3
  Env1 : InportShadow
  Env2 : InportShadow
  FlatEarthToLLA : FlatEarth2LLA  R=6378137
  Ground : Ground
  Manual Switch : ManualSwitch  CurrentSetting=0
  Mux : Mux  Inputs=3
  Product : Product
  Propulsion F,M : Subsystem
  RocketEngineActuators : Subsystem
  Signal Specification : SignalSpecification  Dimensions=[1 3]
  Time Varying Parameters : Subsystem
  PlantData : Outport
  tag scope: sensedAct=global
  wires:
  ActCmd/1 -> RocketEngineActuators/2(Commands)
  RocketEngineActuators/1(Positions) -> Propulsion F,M/1(Actuators)
  Bus Creator/1 -> Aerodynamics/1(Plant), PlantData/1  "PlantData"
  3DOF to 6DOF/2(Xe) -> Bus Creator/5, FlatEarthToLLA/1  "Xe"
  Demux/1 -> Bus Creator/1  "lat"
  Demux/2 -> Bus Creator/2  "long"
  FlatEarthToLLA/1 -> Demux/1
  FlatEarthToLLA/2 -> Bus Creator/3  "alt"
  Ground/1 -> FlatEarthToLLA/2
  3DOF to 6DOF/1(Ve) -> Bus Creator/4  "Ve"
  3DOF to 6DOF/3(phi,theta,psi) -> Demux1/1  "body angles"
  Demux1/1 -> Bus Creator1/1  "phi"
  Demux1/2 -> Bus Creator1/2  "theta"
  Demux1/3 -> Bus Creator1/3  "psi"
  Bus Creator1/1 -> Bus Creator/6  "body angles"
  3DOF to 6DOF/4(DCMbe) -> Bus Creator/7  "DCMbe"
  3DOF to 6DOF/5(Vb) -> Bus Creator/8  "Vb"
  3DOF to 6DOF/6("alpha, beta") -> Demux2/1
  Demux2/1 -> Bus Creator/9  "alpha"
  Demux2/2 -> Bus Creator/10  "beta"
  Demux3/2 -> Bus Creator/12  "beta_dot"
  Demux3/1 -> Bus Creator/11  "alpha_dot"
  3DOF to 6DOF/7("alpha_dot, beta_dot") -> Demux3/1
  3DOF to 6DOF/8(omega) -> Demux4/1  "w"
  3DOF to 6DOF/9(omega_dot) -> Bus Creator/14  "w_dot"
  Signal Specification/1 -> Bus Creator/15  "Ab"
  [pqrWind] -> Bus Creator/16
  [sensedAct] -> Bus Creator/17
  RocketEngineActuators/2(Sensed_Out) -> [sensedAct]
  Aerodynamics/3(pqr_wind) -> [pqrWind]  "pqrWind"
  Propulsion F,M/1(F) -> Add/3  "F_thrust"
  [CG] -> Bus Creator/18  "CG"
  [mass] -> Bus Creator/19  "mass"
  Env1/1 -> Bus Selector/1  "ENV"
  Bus Selector/1 -> Add/1  "<Fg>"
  Env/1 -> Aerodynamics/2(EnvData), RocketEngineActuators/1(ENV)  "ENV"
  Propulsion F,M/2(M) -> Add1/2  "M_thrust"
  Clock/1 -> Time Varying Parameters/1(t)
  Time Varying Parameters/1(dIdt_Tensor(3x3)) -> 3DOF to 6DOF/4(dI/dt)  "dI/dt"
  Time Varying Parameters/2(MOI_Tensor(3x3)) -> 3DOF to 6DOF/5(I)  "I"
  Time Varying Parameters/3(mass) -> [mass]  "mass"
  Time Varying Parameters/4(COM_X) -> [CG]  "CG"
  [mass] -> 3DOF to 6DOF/3(m)
  Add1/1 -> Product/2  "M_total"
  Add/1 -> 3DOF to 6DOF/1(F)  "F_total"
  Aerodynamics/1(F) -> Add/2  "F_aero"
  Env2/1 -> 3DOF to 6DOF/6(Env)  "ENV"
  [CG] -> Propulsion F,M/2(CG)  "CG"
  Aerodynamics/2(M) -> Add1/1  "M_aero"
  3DOF to 6DOF/11(DCMwb) -> Bus Creator/20  "DCMwb"
  Demux4/1 -> Bus Creator2/1  "phi_dot"
  Demux4/3 -> Bus Creator2/3  "psi_dot"
  Demux4/2 -> Bus Creator2/2  "theta_dot"
  Bus Creator2/1 -> Bus Creator/13  "w"
  Demux5/1 -> Mux/1  "Ab_x"
  Demux5/2 -> Mux/2  "Ab_y"
  Demux5/3 -> Mux/3  "Ab_z"
  3DOF to 6DOF/10(Ab) -> Demux5/1  "Ab"
  Mux/1 -> Signal Specification/1  "Ab"
  Clock1/1 -> Compare To Constant/1
  Product/1 -> 3DOF to 6DOF/2(M)
  Compare To Constant/1 -> Manual Switch/1
  Manual Switch/1 -> Product/1
  Constant/1 -> Manual Switch/2

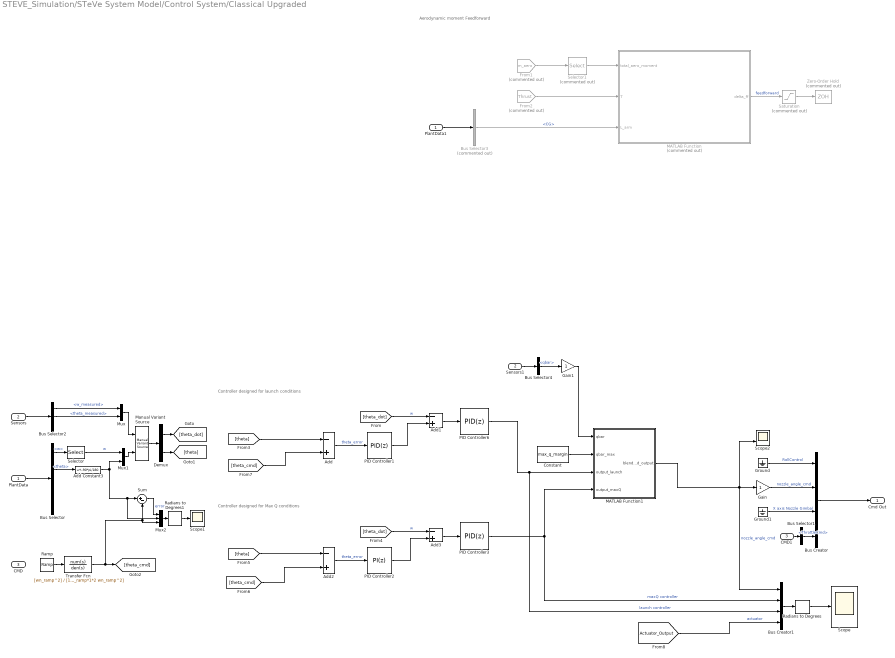
== system STEVE_Simulation/STeVe System Model/Control System/Classical Upgraded ==
  note: Controller designed for launch conditions
  note: Aerodynamic moment Feedforward
  note: Controller designed for Max Q conditions
  PlantData : Inport
  Sensors : Inport  Port=2
  CMD : Inport  Port=3
  Add{,1..3} (4 alike) : Sum  Inputs=-+
  Add Constant3 : Bias  Bias=-90*pi/180  SaturateOnIntegerOverflow=off
  Bus Creator : BusCreator  Inputs=4
  Bus Creator1 : BusCreator  Inputs=4
  Bus Selector : BusSelector  OutputSignals=w,body angles.theta,Ve,Xe
  Bus Selector1 : BusSelector  OutputSignals=ThrottleCmd
  Bus Selector2 : BusSelector  OutputSignals=w_measured,theta_measured,qbar
  Bus Selector3 : BusSelector  Commented=on  OutputSignals=CG
  Bus Selector4 : BusSelector  OutputSignals=qbar
  CMD1 : InportShadow  Port=3
  Constant : Constant  Value=max_q_margin
  Demux : Demux  Outputs=2
  From1 : From  Commented=on  GotoTag=m_aero  TagVisibility=global
  From2 : From  Commented=on  GotoTag=Thrust  TagVisibility=global
  Gain : Gain
  Gain1 : Gain
  Ground : Ground
  Ground1 : Ground
  MATLAB Function : MATLAB Function  Commented=on  TreatAsAtomicUnit=on
  MATLAB Function1 : MATLAB Function  TreatAsAtomicUnit=on
  Manual Variant Source : simulink/Signal Routing/Manual Variant Source  NumChoices=2  LabelModeActiveChoice=V_1
  Mux : Mux  Inputs=2
  Mux1 : Mux  Inputs=2
  Mux2 : Mux  Inputs=3
  PID Controller1 : slpidlib/PID Controller  Controller=PID  Form=Parallel  TimeDomain=Discrete-time  UseExternalTs=off  SampleTime=Ts_outer  IntegratorMethod=Forward Euler  FilterMethod=Forward Euler  ControllerParametersSource=internal  P=C_outer_launch_d_Kp  I=C_outer_launch_d_Ki  UseKiTs=off  D=C_outer_launch_d_Kd  UseExternalDerivativeSource=off  N=C_outer_launch_d_N  UseFilter=on  TunerSelectOption=Transfer Function Based (PID Tuner App)  InitialConditionSource=internal  InitialConditionForIntegrator=0  InitialConditionForFilter=0  DifferentiatorICPrevScaledInput=0  ExternalReset=none  TrackingMode=off  Kt=1  LimitOutput=off  SatLimitsSource=internal  UpperSaturationLimit=inf  LowerSaturationLimit=-inf  LinearizeAsGain=on  AntiWindupMode=none  Kb=1  LimitIntegrator=off  UpperIntegratorSaturationLimit=inf  LowerIntegratorSaturationLimit=-inf  POutMin=[]  POutMax=[]  IOutMin=[]  IOutMax=[]  DOutMin=[]  DOutMax=[]  NOutMin=[]  NOutMax=[]  SumOutMin=[]  SumOutMax=[]  SaturationOutMin=[]  SaturationOutMax=[]  PParamMin=[]  PParamMax=[]  IParamMin=[]  IParamMax=[]  DParamMin=[]  DParamMax=[]  NParamMin=[]  NParamMax=[]  KbParamMin=[]  KbParamMax=[]  KtParamMin=[]  KtParamMax=[]  KbOutMin=[]  KbOutMax=[]  KtOutMin=[]  KtOutMax=[]  IntegratorOutMin=[]  IntegratorOutMax=[]  FilterOutMin=[]  FilterOutMax=[]  SumI1OutMin=[]  SumI1OutMax=[]  SumI2OutMin=[]  SumI2OutMax=[]  SumI3OutMin=[]  SumI3OutMax=[]  SumI4OutMin=[]  SumI4OutMax=[]  SumDOutMin=[]  SumDOutMax=[]  DifferentiatorOutMin=[]  DifferentiatorOutMax=[]  FilterDiffOutCoefMin=[]  FilterDiffOutCoefMax=[]  ReciprocalOutMin=[]  ReciprocalOutMax=[]  SumDenOutMin=[]  SumDenOutMax=[]  SumNumOutMin=[]  SumNumOutMax=[]  DivideOutMin=[]  DivideOutMax=[]  UdiffTsProdOutMin=[]  UdiffTsProdOutMax=[]  NTsProdOutMin=[]  NTsProdOutMax=[]  UintegralTsProdOutMin=[]  UintegralTsProdOutMax=[]  UngainTsProdOutMin=[]  UngainTsProdOutMax=[]  ClampingZeroOutDataTypeStr=Inherit: Inherit via back propagation  ClampingZeroOutMin=[]  ClampingZeroOutMax=[]  FilterDenConstantOutDataTypeStr=Inherit: Inherit via back propagation  FilterDenConstantOutMin=[]  FilterDenConstantOutMax=[]  PCopyOutDataTypeStr=Inherit: Inherit via back propagation  PCopyOutMin=[]  PCopyOutMax=[]  NCopyOutDataTypeStr=Inherit: Inherit via back propagation  NCopyOutMin=[]  NCopyOutMax=[]  IntegratorContinuousStateAttributes=''  IntegratorStateMustResolveToSignalObject=off  IntegratorRTWStateStorageClass=Auto  FilterContinuousStateAttributes=''  FilterStateMustResolveToSignalObject=off  FilterRTWStateStorageClass=Auto  ParallelPVariant=InternalParameters  IdealPVariant=Disabled  IVariant=InternalParameters  DVariant=InternalParameters  IntegratorVariant=Discrete  SatVariant=Disabled  AWVariant=Passthrough  PCopyVariant=Disabled  TRVariant=Disabled  FdbkBlocksVariant=Forward  IdealPFdbkVariant=Disabled  SatFdbkVariant=Disabled  DerivativeFilterVariant=ForwardEulerFilter  NVariant=InternalParameters  NCopyVariant=Disabled  FilterICVariant=InternalICsFilter  IntegratorICVariant=InternalICs  ExternalResetVariant=Disabled  TRSumVariant=Passthrough  SumFdbkVariant=Disabled  SumVariant=Sum_PID  TsampFilterVariant=InternalTs  TsampNgainVariant=Passthrough  TsampIntegralVariant=Disabled_SignalSpec  ExternalSaturationOutDataTypeStr=Inherit: Same as second input  DerivativeSourceVariant=ErrorSignal  PreIntVariant=InternalPreInt
  PID Controller2 : slpidlib/PID Controller  Controller=PI  Form=Parallel  TimeDomain=Discrete-time  UseExternalTs=off  SampleTime=Ts_outer  IntegratorMethod=Forward Euler  FilterMethod=Forward Euler  ControllerParametersSource=internal  P=C_outer_maxQ_d_Kp  I=C_outer_maxQ_d_Ki  UseKiTs=off  D=C_outer_maxQ_d_Kd  UseExternalDerivativeSource=off  N=3.44088549948957  UseFilter=off  TunerSelectOption=Transfer Function Based (PID Tuner App)  InitialConditionSource=internal  InitialConditionForIntegrator=0  InitialConditionForFilter=0  DifferentiatorICPrevScaledInput=0  ExternalReset=none  TrackingMode=off  Kt=1  LimitOutput=off  SatLimitsSource=internal  UpperSaturationLimit=inf  LowerSaturationLimit=-inf  LinearizeAsGain=on  AntiWindupMode=none  Kb=1  LimitIntegrator=off  UpperIntegratorSaturationLimit=inf  LowerIntegratorSaturationLimit=-inf  POutMin=[]  POutMax=[]  IOutMin=[]  IOutMax=[]  DOutMin=[]  DOutMax=[]  NOutMin=[]  NOutMax=[]  SumOutMin=[]  SumOutMax=[]  SaturationOutMin=[]  SaturationOutMax=[]  PParamMin=[]  PParamMax=[]  IParamMin=[]  IParamMax=[]  DParamMin=[]  DParamMax=[]  NParamMin=[]  NParamMax=[]  KbParamMin=[]  KbParamMax=[]  KtParamMin=[]  KtParamMax=[]  KbOutMin=[]  KbOutMax=[]  KtOutMin=[]  KtOutMax=[]  IntegratorOutMin=[]  IntegratorOutMax=[]  FilterOutMin=[]  FilterOutMax=[]  SumI1OutMin=[]  SumI1OutMax=[]  SumI2OutMin=[]  SumI2OutMax=[]  SumI3OutMin=[]  SumI3OutMax=[]  SumI4OutMin=[]  SumI4OutMax=[]  SumDOutMin=[]  SumDOutMax=[]  DifferentiatorOutMin=[]  DifferentiatorOutMax=[]  FilterDiffOutCoefMin=[]  FilterDiffOutCoefMax=[]  ReciprocalOutMin=[]  ReciprocalOutMax=[]  SumDenOutMin=[]  SumDenOutMax=[]  SumNumOutMin=[]  SumNumOutMax=[]  DivideOutMin=[]  DivideOutMax=[]  UdiffTsProdOutMin=[]  UdiffTsProdOutMax=[]  NTsProdOutMin=[]  NTsProdOutMax=[]  UintegralTsProdOutMin=[]  UintegralTsProdOutMax=[]  UngainTsProdOutMin=[]  UngainTsProdOutMax=[]  ClampingZeroOutDataTypeStr=Inherit: Inherit via back propagation  ClampingZeroOutMin=[]  ClampingZeroOutMax=[]  FilterDenConstantOutDataTypeStr=Inherit: Inherit via back propagation  FilterDenConstantOutMin=[]  FilterDenConstantOutMax=[]  PCopyOutDataTypeStr=Inherit: Inherit via back propagation  PCopyOutMin=[]  PCopyOutMax=[]  NCopyOutDataTypeStr=Inherit: Inherit via back propagation  NCopyOutMin=[]  NCopyOutMax=[]  IntegratorContinuousStateAttributes=''  IntegratorStateMustResolveToSignalObject=off  IntegratorRTWStateStorageClass=Auto  FilterContinuousStateAttributes=''  FilterStateMustResolveToSignalObject=off  FilterRTWStateStorageClass=Auto  ParallelPVariant=InternalParameters  IdealPVariant=Disabled  IVariant=InternalParameters  DVariant=Disabled  IntegratorVariant=Discrete  SatVariant=Disabled  AWVariant=Passthrough  PCopyVariant=Disabled  TRVariant=Disabled  FdbkBlocksVariant=Forward  IdealPFdbkVariant=Disabled  SatFdbkVariant=Disabled  DerivativeFilterVariant=Disabled  NVariant=Disabled  NCopyVariant=Disabled_SignalSpec  FilterICVariant=Disabled  IntegratorICVariant=InternalICs  ExternalResetVariant=Disabled  TRSumVariant=Passthrough  SumFdbkVariant=Disabled  SumVariant=Sum_PI  TsampFilterVariant=InternalTs  TsampNgainVariant=Passthrough  TsampIntegralVariant=Disabled_SignalSpec  ExternalSaturationOutDataTypeStr=Inherit: Same as second input  DerivativeSourceVariant=Disabled  PreIntVariant=InternalPreInt
  PID Controller3 : slpidlib/PID Controller  Controller=PID  Form=Parallel  TimeDomain=Discrete-time  UseExternalTs=off  SampleTime=Ts_inner  IntegratorMethod=Forward Euler  FilterMethod=Forward Euler  ControllerParametersSource=internal  P=C_inner_maxQ_d_Kp  I=C_inner_maxQ_d_Ki  UseKiTs=off  D=C_inner_maxQ_d_Kd  UseExternalDerivativeSource=off  N=C_inner_maxQ_d_Tf  UseFilter=on  TunerSelectOption=Transfer Function Based (PID Tuner App)  InitialConditionSource=internal  InitialConditionForIntegrator=0  InitialConditionForFilter=0  DifferentiatorICPrevScaledInput=0  ExternalReset=none  TrackingMode=off  Kt=1  LimitOutput=on  SatLimitsSource=internal  UpperSaturationLimit=10*pi/180  LowerSaturationLimit=-10*pi/180  LinearizeAsGain=on  AntiWindupMode=clamping  Kb=1  LimitIntegrator=on  UpperIntegratorSaturationLimit=10*pi/180  LowerIntegratorSaturationLimit=-10*pi/180  POutMin=[]  POutMax=[]  IOutMin=[]  IOutMax=[]  DOutMin=[]  DOutMax=[]  NOutMin=[]  NOutMax=[]  SumOutMin=[]  SumOutMax=[]  SaturationOutMin=[]  SaturationOutMax=[]  PParamMin=[]  PParamMax=[]  IParamMin=[]  IParamMax=[]  DParamMin=[]  DParamMax=[]  NParamMin=[]  NParamMax=[]  KbParamMin=[]  KbParamMax=[]  KtParamMin=[]  KtParamMax=[]  KbOutMin=[]  KbOutMax=[]  KtOutMin=[]  KtOutMax=[]  IntegratorOutMin=[]  IntegratorOutMax=[]  FilterOutMin=[]  FilterOutMax=[]  SumI1OutMin=[]  SumI1OutMax=[]  SumI2OutMin=[]  SumI2OutMax=[]  SumI3OutMin=[]  SumI3OutMax=[]  SumI4OutMin=[]  SumI4OutMax=[]  SumDOutMin=[]  SumDOutMax=[]  DifferentiatorOutMin=[]  DifferentiatorOutMax=[]  FilterDiffOutCoefMin=[]  FilterDiffOutCoefMax=[]  ReciprocalOutMin=[]  ReciprocalOutMax=[]  SumDenOutMin=[]  SumDenOutMax=[]  SumNumOutMin=[]  SumNumOutMax=[]  DivideOutMin=[]  DivideOutMax=[]  UdiffTsProdOutMin=[]  UdiffTsProdOutMax=[]  NTsProdOutMin=[]  NTsProdOutMax=[]  UintegralTsProdOutMin=[]  UintegralTsProdOutMax=[]  UngainTsProdOutMin=[]  UngainTsProdOutMax=[]  ClampingZeroOutDataTypeStr=Inherit: Inherit via back propagation  ClampingZeroOutMin=[]  ClampingZeroOutMax=[]  FilterDenConstantOutDataTypeStr=Inherit: Inherit via back propagation  FilterDenConstantOutMin=[]  FilterDenConstantOutMax=[]  PCopyOutDataTypeStr=Inherit: Inherit via back propagation  PCopyOutMin=[]  PCopyOutMax=[]  NCopyOutDataTypeStr=Inherit: Inherit via back propagation  NCopyOutMin=[]  NCopyOutMax=[]  IntegratorContinuousStateAttributes=''  IntegratorStateMustResolveToSignalObject=off  IntegratorRTWStateStorageClass=Auto  FilterContinuousStateAttributes=''  FilterStateMustResolveToSignalObject=off  FilterRTWStateStorageClass=Auto  ParallelPVariant=InternalParameters  IdealPVariant=Disabled  IVariant=InternalParameters  DVariant=InternalParameters  IntegratorVariant=Discrete  SatVariant=Enabled  AWVariant=DiscClampingParallel  PCopyVariant=Disabled  TRVariant=Disabled  FdbkBlocksVariant=Forward  IdealPFdbkVariant=Disabled  SatFdbkVariant=Disabled  DerivativeFilterVariant=ForwardEulerFilter  NVariant=InternalParameters  NCopyVariant=Disabled  FilterICVariant=InternalICsFilter  IntegratorICVariant=InternalICs  ExternalResetVariant=Disabled  TRSumVariant=Passthrough  SumFdbkVariant=Disabled  SumVariant=Sum_PID  TsampFilterVariant=InternalTs  TsampNgainVariant=Passthrough  TsampIntegralVariant=Disabled_SignalSpec  ExternalSaturationOutDataTypeStr=Inherit: Same as second input  DerivativeSourceVariant=ErrorSignal  PreIntVariant=InternalPreInt
  PID Controller6 : slpidlib/PID Controller  Controller=PID  Form=Parallel  TimeDomain=Discrete-time  UseExternalTs=off  SampleTime=Ts_inner  IntegratorMethod=Forward Euler  FilterMethod=Forward Euler  ControllerParametersSource=internal  P=C_inner_launch_d_Kp  I=C_inner_launch_d_Ki  UseKiTs=off  D=C_inner_launch_d_Kd  UseExternalDerivativeSource=off  N=100  UseFilter=off  TunerSelectOption=Transfer Function Based (PID Tuner App)  InitialConditionSource=internal  InitialConditionForIntegrator=0  InitialConditionForFilter=0  DifferentiatorICPrevScaledInput=0  ExternalReset=none  TrackingMode=off  Kt=1  LimitOutput=on  SatLimitsSource=internal  UpperSaturationLimit=10*pi/180  LowerSaturationLimit=-10*pi/180  LinearizeAsGain=on  AntiWindupMode=clamping  Kb=1  LimitIntegrator=on  UpperIntegratorSaturationLimit=10*pi/180  LowerIntegratorSaturationLimit=-10*pi/180  POutMin=[]  POutMax=[]  IOutMin=[]  IOutMax=[]  DOutMin=[]  DOutMax=[]  NOutMin=[]  NOutMax=[]  SumOutMin=[]  SumOutMax=[]  SaturationOutMin=[]  SaturationOutMax=[]  PParamMin=[]  PParamMax=[]  IParamMin=[]  IParamMax=[]  DParamMin=[]  DParamMax=[]  NParamMin=[]  NParamMax=[]  KbParamMin=[]  KbParamMax=[]  KtParamMin=[]  KtParamMax=[]  KbOutMin=[]  KbOutMax=[]  KtOutMin=[]  KtOutMax=[]  IntegratorOutMin=[]  IntegratorOutMax=[]  FilterOutMin=[]  FilterOutMax=[]  SumI1OutMin=[]  SumI1OutMax=[]  SumI2OutMin=[]  SumI2OutMax=[]  SumI3OutMin=[]  SumI3OutMax=[]  SumI4OutMin=[]  SumI4OutMax=[]  SumDOutMin=[]  SumDOutMax=[]  DifferentiatorOutMin=[]  DifferentiatorOutMax=[]  FilterDiffOutCoefMin=[]  FilterDiffOutCoefMax=[]  ReciprocalOutMin=[]  ReciprocalOutMax=[]  SumDenOutMin=[]  SumDenOutMax=[]  SumNumOutMin=[]  SumNumOutMax=[]  DivideOutMin=[]  DivideOutMax=[]  UdiffTsProdOutMin=[]  UdiffTsProdOutMax=[]  NTsProdOutMin=[]  NTsProdOutMax=[]  UintegralTsProdOutMin=[]  UintegralTsProdOutMax=[]  UngainTsProdOutMin=[]  UngainTsProdOutMax=[]  ClampingZeroOutDataTypeStr=Inherit: Inherit via back propagation  ClampingZeroOutMin=[]  ClampingZeroOutMax=[]  FilterDenConstantOutDataTypeStr=Inherit: Inherit via back propagation  FilterDenConstantOutMin=[]  FilterDenConstantOutMax=[]  PCopyOutDataTypeStr=Inherit: Inherit via back propagation  PCopyOutMin=[]  PCopyOutMax=[]  NCopyOutDataTypeStr=Inherit: Inherit via back propagation  NCopyOutMin=[]  NCopyOutMax=[]  IntegratorContinuousStateAttributes=''  IntegratorStateMustResolveToSignalObject=off  IntegratorRTWStateStorageClass=Auto  FilterContinuousStateAttributes=''  FilterStateMustResolveToSignalObject=off  FilterRTWStateStorageClass=Auto  ParallelPVariant=InternalParameters  IdealPVariant=Disabled  IVariant=InternalParameters  DVariant=InternalParameters  IntegratorVariant=Discrete  SatVariant=Enabled  AWVariant=DiscClampingParallel  PCopyVariant=Disabled  TRVariant=Disabled  FdbkBlocksVariant=Forward  IdealPFdbkVariant=Disabled  SatFdbkVariant=Disabled  DerivativeFilterVariant=Differentiator  NVariant=Passthrough  NCopyVariant=Disabled_SignalSpec  FilterICVariant=InternalICsDifferentiator  IntegratorICVariant=InternalICs  ExternalResetVariant=Disabled  TRSumVariant=Passthrough  SumFdbkVariant=Disabled  SumVariant=Sum_PID  TsampFilterVariant=InternalTs  TsampNgainVariant=Passthrough  TsampIntegralVariant=Disabled_SignalSpec  ExternalSaturationOutDataTypeStr=Inherit: Same as second input  DerivativeSourceVariant=ErrorSignal  PreIntVariant=InternalPreInt
  PlantData1 : InportShadow
  Radians to Degrees : simulink_extras/Transformations/Radians to Degrees
  Radians to Degrees1 : simulink_extras/Transformations/Radians to Degrees
  Ramp : simulink/Sources/Ramp  slope=-(50/60)*pi/180  start=0  InitialOutput=0
  Saturation : Saturate  Commented=on  UpperLimit=10*pi/180  LowerLimit=-10*pi/180
  Scope : Scope
      settings: ActiveDisplayYMinimum=-0.083485750616447252  ActiveDisplayYMaximum=2.7048040540539371  DataLoggingVariableName=ScopeData3
  Scope1 : Scope
      settings: ActiveDisplayYMinimum=-44.397461498284216  ActiveDisplayYMaximum=2.337544107445984  DataLoggingVariableName=ScopeData4
  Scope2 : Scope  NumInputPorts=2
      settings: ActiveDisplayYMinimum=0.00039650314567646317  ActiveDisplayYMaximum=0.0024847856778169785  DataLoggingVariableName=ScopeData9
  Selector : Selector  InputPortWidth=3  IndexOptions=Index vector (dialog)  Indices=[2]  OutputSizes=1
  Selector1 : Selector  Commented=on  InputPortWidth=3  IndexOptions=Index vector (dialog)  Indices=[2]  OutputSizes=1
  Sensors1 : InportShadow  Port=2
  Sum : Sum  Inputs=|+-
  Transfer Fcn : TransferFcn  Numerator=[wn_ramp^2]  Denominator=[1 wn_ramp*1*2 wn_ramp^2]
  Zero-Order Hold : ZeroOrderHold  Commented=on  SampleTime=0.005
  Cmd Out : Outport
  wires:
  Selector1/1 -> MATLAB Function/1(total_aero_moment)
  PlantData/1 -> Bus Selector/1
  From1/1 -> Selector1/1
  Bus Selector/1 -> Selector/1  "<w>"
  Ground1/1 -> Bus Creator/3  "X axis Nozzle Gimbal"
  Bus Selector3/1 -> MATLAB Function/3(L_arm)  "<CG>"
  Gain/1 -> Bus Creator/2  "nozzle_angle_cmd"
  MATLAB Function/1(delta_ff) -> Saturation/1  "feedforward"
  [theta_dot] -> Add1/1  "w"
  PlantData1/1 -> Bus Selector3/1
  [theta_cmd] -> Add/2
  Ground/1 -> Bus Creator/1  "RollControl"
  From2/1 -> MATLAB Function/2(T)
  Bus Creator/1 -> Cmd Out/1
  Add/1 -> PID Controller1/1  "theta_error"
  PID Controller6/1 -> Bus Creator1/3, MATLAB Function1/3(output_launch)  "launch controller"
  Add1/1 -> PID Controller6/1
  Sensors/1 -> Bus Selector2/1
  Saturation/1 -> Zero-Order Hold/1
  [theta] -> Add/1
  CMD1/1 -> Bus Selector1/1
  Bus Selector1/1 -> Bus Creator/4  "<ThrottleCmd>"
  PID Controller1/1 -> Add1/2
  Bus Selector/2 -> Add Constant3/1  "<theta>"
  Add2/1 -> PID Controller2/1  "theta_error"
  [theta] -> Add2/1
  Add3/1 -> PID Controller3/1
  PID Controller3/1 -> Bus Creator1/2, MATLAB Function1/4(output_maxQ)  "maxQ controller"
  PID Controller2/1 -> Add3/2
  [theta_cmd] -> Add2/2
  [theta_dot] -> Add3/1  "w"
  Ramp/1 -> Transfer Fcn/1
  Sensors1/1 -> Bus Selector4/1
  MATLAB Function1/1(blended_output) -> Bus Creator1/1, Scope2/2, Gain/1  "nozzle_angle_cmd"
  Constant/1 -> MATLAB Function1/2(qbar_max)
  Bus Selector4/1 -> Gain1/1  "<qbar>"
  [Actuator_Output] -> Bus Creator1/4  "actuator"
  Transfer Fcn/1 -> Mux2/3, Sum/2, [theta_cmd]
  Bus Selector2/1 -> Mux/1  "<w_measured>"
  Bus Selector2/2 -> Mux/2  "<theta_measured>"
  Mux/1 -> Manual Variant Source/1
  Manual Variant Source/1 -> Demux/1
  Demux/1 -> [theta_dot]
  Demux/2 -> [theta]
  Selector/1 -> Mux1/1  "w"
  Mux1/1 -> Manual Variant Source/2
  Add Constant3/1 -> Mux2/2, Sum/1, Mux1/2
  Sum/1 -> Mux2/1  "error"
  Gain1/1 -> MATLAB Function1/1(qbar)
  Bus Creator1/1 -> Radians to Degrees/1
  Radians to Degrees/1 -> Scope/1
  Mux2/1 -> Radians to Degrees1/1
  Radians to Degrees1/1 -> Scope1/1

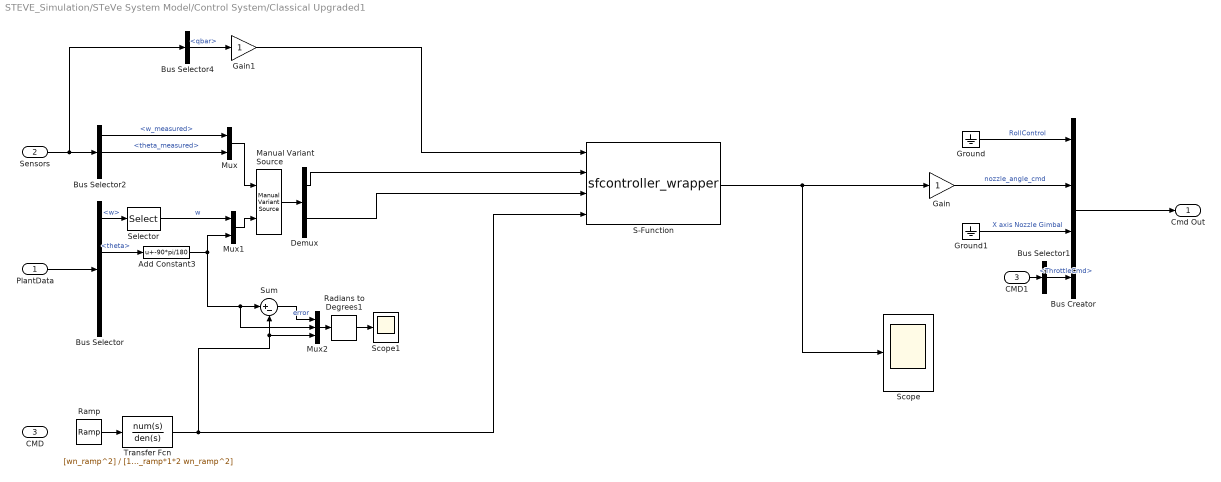
== system STEVE_Simulation/STeVe System Model/Control System/Classical Upgraded1 ==
  PlantData : Inport
  Sensors : Inport  Port=2
  CMD : Inport  Port=3
  Add Constant3 : Bias  Bias=-90*pi/180  SaturateOnIntegerOverflow=off
  Bus Creator : BusCreator  Inputs=4
  Bus Selector : BusSelector  OutputSignals=w,body angles.theta,Ve,Xe
  Bus Selector1 : BusSelector  OutputSignals=ThrottleCmd
  Bus Selector2 : BusSelector  OutputSignals=w_measured,theta_measured,qbar
  Bus Selector4 : BusSelector  OutputSignals=qbar
  CMD1 : InportShadow  Port=3
  Demux : Demux  Outputs=2
  Gain : Gain
  Gain1 : Gain
  Ground : Ground
  Ground1 : Ground
  Manual Variant Source : simulink/Signal Routing/Manual Variant Source  NumChoices=2  LabelModeActiveChoice=V_2
  Mux : Mux  Inputs=2
  Mux1 : Mux  Inputs=2
  Mux2 : Mux  Inputs=3
  Radians to Degrees1 : simulink_extras/Transformations/Radians to Degrees
  Ramp : simulink/Sources/Ramp  slope=-(10/60)*pi/180  start=0  InitialOutput=0
  S-Function : S-Function  FunctionName=sfcontroller_wrapper  Parameters=1/200  SFunctionDeploymentMode=off  EnableBusSupport=off
  Scope : Scope
      settings: ActiveDisplayYMinimum=-0.0062156776996311752  ActiveDisplayYMaximum=0.042555941250627768  DataLoggingVariableName=ScopeData3
  Scope1 : Scope
      settings: ActiveDisplayYMinimum=-44.397461498284216  ActiveDisplayYMaximum=2.337544107445984  DataLoggingVariableName=ScopeData4
  Selector : Selector  InputPortWidth=3  IndexOptions=Index vector (dialog)  Indices=[2]  OutputSizes=1
  Sum : Sum  Inputs=|+-
  Transfer Fcn : TransferFcn  Numerator=[wn_ramp^2]  Denominator=[1 wn_ramp*1*2 wn_ramp^2]
  Cmd Out : Outport
  wires:
  PlantData/1 -> Bus Selector/1
  Bus Selector/1 -> Selector/1  "<w>"
  Ground1/1 -> Bus Creator/3  "X axis Nozzle Gimbal"
  Gain/1 -> Bus Creator/2  "nozzle_angle_cmd"
  Ground/1 -> Bus Creator/1  "RollControl"
  Bus Creator/1 -> Cmd Out/1
  CMD1/1 -> Bus Selector1/1
  Bus Selector1/1 -> Bus Creator/4  "<ThrottleCmd>"
  Bus Selector/2 -> Add Constant3/1  "<theta>"
  Ramp/1 -> Transfer Fcn/1
  Transfer Fcn/1 -> S-Function/4, Mux2/3, Sum/2
  Bus Selector2/1 -> Mux/1  "<w_measured>"
  Bus Selector2/2 -> Mux/2  "<theta_measured>"
  Mux/1 -> Manual Variant Source/1
  Manual Variant Source/1 -> Demux/1
  Demux/1 -> S-Function/2
  Demux/2 -> S-Function/3
  Selector/1 -> Mux1/1  "w"
  Mux1/1 -> Manual Variant Source/2
  Add Constant3/1 -> Mux2/2, Sum/1, Mux1/2
  Sum/1 -> Mux2/1  "error"
  Mux2/1 -> Radians to Degrees1/1
  Radians to Degrees1/1 -> Scope1/1
  Sensors/1 -> Bus Selector4/1, Bus Selector2/1
  Bus Selector4/1 -> Gain1/1  "<qbar>"
  S-Function/1 -> Scope/1, Gain/1
  Gain1/1 -> S-Function/1
